simulink model "pendSimPID"  (R2024b)
settings: Solver=FixedStepAuto  StartTime=0.0  StopTime=1.3  FixedStep=0.001  MaxStep=0.005  RelTol=1e-3
settings Model: Creator=mattf  LastModifiedBy=nicholas

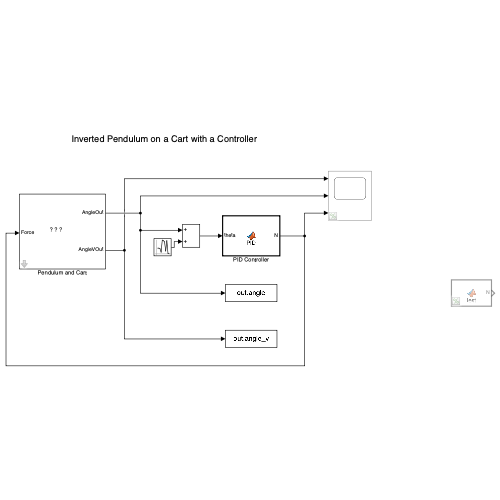
[thumbnail: Simulink's stored preview of the top-level diagram]
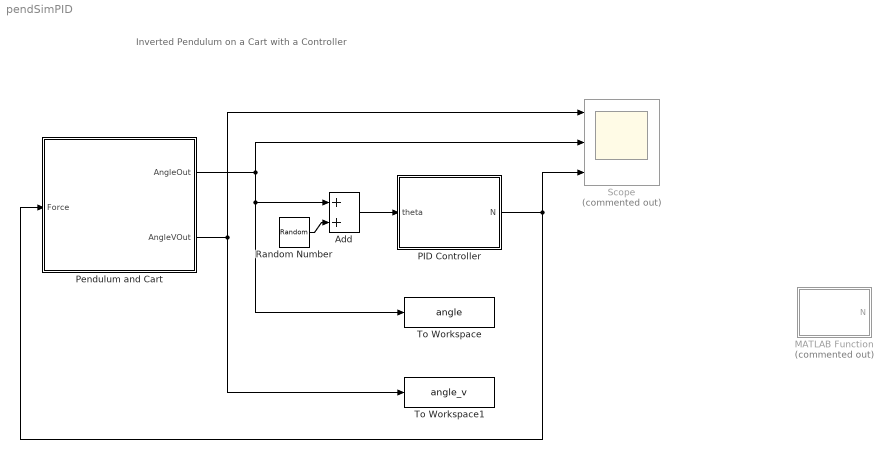
== system pendSimPID ==
  note: Inverted Pendulum on a Cart with a Controller
  Add : Sum
  MATLAB Function : MATLAB Function  Commented=on  TreatAsAtomicUnit=on
  PID Controller : MATLAB Function  TreatAsAtomicUnit=on
  Pendulum and Cart : Subsystem  mask{Mcart=0.5, m=0.2, l=0.3/2, g=9.8, init=pi/6}
      mask prompts: Mcart "Cart Mass (kg):"; m "Pend Mass (kg):"; l "COM Distance (m):"; g "Acc due to Gravity (g):"; init "Initial Angle (rad):"
      mask Display: image('pen img.png');
  Random Number : RandomNumber  SampleTime=0.001
  Scope : Scope  Commented=on  NumInputPorts=3
  To Workspace : ToWorkspace  VariableName=angle  SampleTime=-1
  To Workspace1 : ToWorkspace  VariableName=angle_v  SampleTime=-1
  wires:
  Pendulum and Cart/2(AngleVOut) -> To Workspace1/1, Scope/1
  Pendulum and Cart/1(AngleOut) -> Add/1, To Workspace/1, Scope/2
  Add/1 -> PID Controller/1(theta)
  PID Controller/1(N) -> Scope/3, Pendulum and Cart/1(Force)
  Random Number/1 -> Add/2

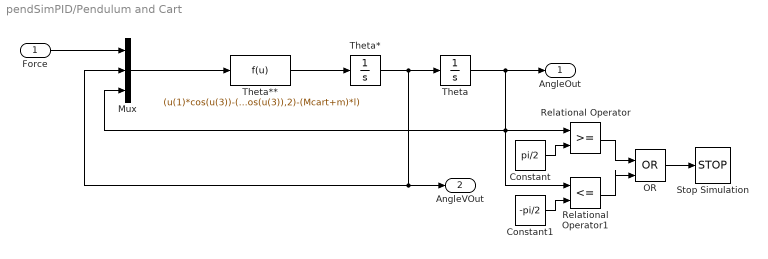
== system pendSimPID/Pendulum and Cart ==
  Force : Inport
  Constant : Constant  Value=pi/2
  Constant1 : Constant  Value=-pi/2
  Mux : Mux  Inputs=3
  OR : Logic  Operator=OR  IconShape=distinctive  AllPortsSameDT=off  OutDataTypeStr=boolean
  Relational Operator : RelationalOperator  OutDataTypeStr=boolean  RndMeth=Simplest  InputSameDT=off
  Relational Operator1 : RelationalOperator  Operator=<=  OutDataTypeStr=boolean  RndMeth=Simplest  InputSameDT=off
  Stop Simulation : Stop
  Theta : Integrator  InitialCondition=init
  Theta* : Integrator
  Theta** : Fcn  Expr=(u(1)*cos(u(3))-(Mcart+m)*g*sin(u(3))+m*l*cos(u(3))*sin(u(3))*power(u(2),2))/(m*l*power(cos(u(3)),2)-(Mcart+m)*l)
  AngleOut : Outport
  AngleVOut : Outport  Port=2
  wires:
  Constant/1 -> Relational Operator/2
  Relational Operator/1 -> OR/1
  Mux/1 -> Theta**/1
  OR/1 -> Stop Simulation/1
  Force/1 -> Mux/1
  Theta**/1 -> Theta*/1
  Constant1/1 -> Relational Operator1/2
  Theta*/1 -> Mux/2, AngleVOut/1, Theta/1
  Theta/1 -> AngleOut/1, Relational Operator1/1, Relational Operator/1, Mux/3
  Relational Operator1/1 -> OR/2

== matlab function pendSimPID/PID Controller ==
  settings: updateMethod=DISCRETE
  data: N output; theta input
function N = PID(theta)

    % call extrinsic python function
    coder.extrinsic('py.PIDControllerPend.controller_call');

    % Call Python function and return result
    N = coder.nullcopy(zeros(1,1)); % no clue why, but this is need.
    N = double(py.PIDControllerPend.controller_call(theta));
    end

== matlab function pendSimPID/MATLAB Function ==
  data: N output
function N = test()
    coder.extrinsic('py.troubleshoot.test');

    N = double(py.troubleshoot.test());
